simulink model "claw_machine_design_sofia"  (R2022b)
settings: Solver=VariableStepAuto  StartTime=0.0  StopTime=inf  RelTol=1e-3
libraries: vrlib x1
settings Model: Creator=Sofia  LastModifiedBy=Sofia

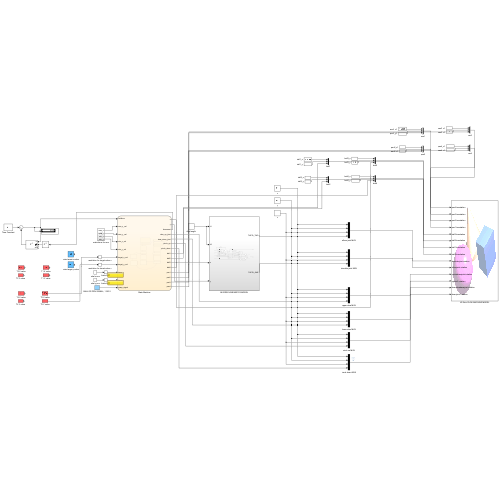
[thumbnail: Simulink's stored preview of the top-level diagram]
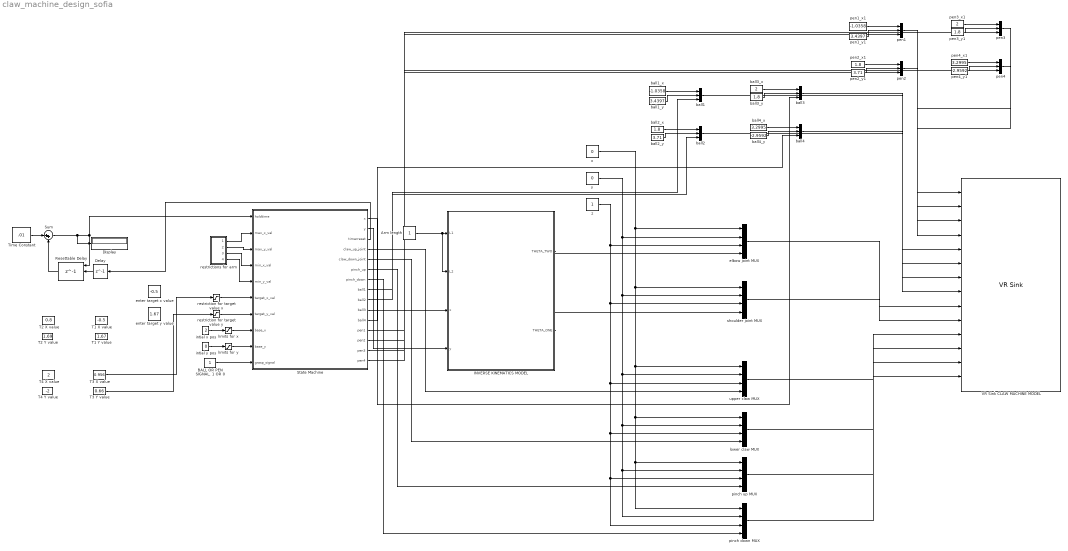
== system claw_machine_design_sofia ==
  Arm length : Constant
  "BALL OR PEN SIGNAL, 1 OR 0" : Constant
  Delay : Delay  DelayLength=1  InitialCondition=0
  Display : Display
  INVERSE KINEMATICS MODEL : Subsystem  Description=Calculates joint angles based on end effector x and y positions
  Resettable Delay : Delay  DelayLength=1  InitialConditionSource=Input port  ExternalReset=Rising
      settings: InputPortMap=u0,r5,p4
  State Machine : Stateflow chart  TreatAsAtomicUnit=on
  Sum : Sum  Inputs=|++
  T1 X value : Constant  Value=-0.5
  T1 Y value : Constant  Value=1.67
  T2 X value : Constant  Value=0.8
  T2 Y value : Constant  Value=1.69
  T3 X value : Constant  Value=0.956
  T3 Y value : Constant  Value=0.66
  T4 X value : Constant  Value=2
  T4 Y value : Constant  Value=-2
  Time Constant : Constant  Value=.01
  VR Sink CLAW MACHINE MODEL : vrlib/VR Sink  InstantiateOnLoad=on  SampleTime=0.1  ViewEnable=on  RemoteChange=off  RemoteView=off  FieldsWritten=pen4.translation.3.1.1.double#pen3.translation.3.1.1.double#pen2.translation.3.1.1.double#pen1.translation.3.1.1.double#ball3.translation.3.1.1.double#ball2.translation.3.1.1.double#ball1.translation.3.1.1.double#ball4.translation.3.1.1.double#shoulderjoint.rotation.4.1.1.double#elbowjoint.rotation.4.1.1.double#upclawbasejoint.rotation.4.1.1.double#upjoint1.rotation.4.1.1.double#downclawbasejoint.rotation.4.1.1.double#downjoint1.rotation.4.1.1.double  WorldFileName=C:\Users\Sofia\OneDrive\Semester 4\691 Brain Computer Interfaces\FINAL PROJECT BCI\clawmachinemodel.wrl  AutoView=off  VideoDimensions=[]  AllowVariableSize=off
  ball{1..4} (4 alike) : Mux  Inputs=3
  ball1_x : Constant  Value=-1.0358
  ball1_y : Constant  Value=3.4397
  ball2_x : Constant  Value=1.8
  ball2_y : Constant  Value=3.71
  ball3_x : Constant  Value=2
  ball3_y : Constant  Value=1.8
  ball4_x : Constant  Value=3.2995
  ball4_y : Constant  Value=-2.9592
  elbow joint MUX : Mux
  enter target x value : Constant  Value=-0.5
  enter target y value : Constant  Value=1.67
  intial x pos : Constant  Value=2
  intial y pos : Constant  Value=0
  limits for x : Saturate  UpperLimit=2  LowerLimit=0
  limits for y : Saturate  UpperLimit=2  LowerLimit=0
  lower claw MUX : Mux
  pen{1..4} (4 alike) : Mux  Inputs=3
  pen1_x1 : Constant  Value=-1.0358
  pen1_y1 : Constant  Value=3.4397
  pen2_x1 : Constant  Value=1.8
  pen2_y1 : Constant  Value=3.71
  pen3_x1 : Constant  Value=2
  pen3_y1 : Constant  Value=1.8
  pen4_x1 : Constant  Value=3.2995
  pen4_y1 : Constant  Value=-2.9592
  pinch down MUX : Mux
  pinch up MUX : Mux
  restriction for target value x : Saturate  UpperLimit=2
  restriction for target value y : Saturate  UpperLimit=2  LowerLimit=-2
  restrictions for arm : Subsystem
  shoulder joint MUX : Mux
  upper claw MUX : Mux
  x : Constant  Value=0
  y : Constant  Value=0
  z : Constant
  wires:
  State Machine/3(timerreset) -> Delay/1
  Resettable Delay/1 -> Sum/2
  x/1 -> shoulder joint MUX/1, upper claw MUX/1, lower claw MUX/1, pinch up MUX/1, pinch down MUX/1, elbow joint MUX/1
  z/1 -> elbow joint MUX/3, shoulder joint MUX/3, upper claw MUX/3, pinch down MUX/3, pinch up MUX/3, lower claw MUX/3
  y/1 -> elbow joint MUX/2, shoulder joint MUX/2, upper claw MUX/2, pinch up MUX/2, pinch down MUX/2, lower claw MUX/2
  Sum/1 -> State Machine/1(holdtime), Resettable Delay/1, Display/1
  Time Constant/1 -> Sum/1
  Delay/1 -> Resettable Delay/2
  Arm length/1 -> INVERSE KINEMATICS MODEL/2(L2), INVERSE KINEMATICS MODEL/1(L1)
  INVERSE KINEMATICS MODEL/2(THETA_ONE) -> shoulder joint MUX/4
  INVERSE KINEMATICS MODEL/1(THETA_TWO) -> elbow joint MUX/4
  State Machine/1(x) -> INVERSE KINEMATICS MODEL/3(x)
  State Machine/2(y) -> INVERSE KINEMATICS MODEL/4(y)
  restrictions for arm/1(max_x) -> State Machine/2(max_x_val)
  restrictions for arm/2(max_y) -> State Machine/3(max_y_val)
  restrictions for arm/3(min_x) -> State Machine/4(min_x_val)
  restrictions for arm/4(min_y) -> State Machine/5(min_y_val)
  restriction for target value x/1 -> State Machine/6(target_x_val)
  restriction for target value y/1 -> State Machine/7(target_y_val)
  "BALL OR PEN SIGNAL, 1 OR 0"/1 -> State Machine/10(grasp_signal)
  ball4_x/1 -> ball4/1
  ball4_y/1 -> ball4/2
  ball1_x/1 -> ball1/1
  ball1_y/1 -> ball1/2
  ball3_x/1 -> ball3/1
  ball3_y/1 -> ball3/2
  ball2_y/1 -> ball2/2
  ball2_x/1 -> ball2/1
  State Machine/4(claw_up_joint) -> upper claw MUX/4
  State Machine/5(claw_down_joint) -> lower claw MUX/4
  State Machine/6(pinch_up) -> pinch up MUX/4
  State Machine/7(pinch_down) -> pinch down MUX/4
  State Machine/8(ball1) -> ball1/3
  State Machine/9(ball2) -> ball2/3
  State Machine/10(ball3) -> ball3/3
  State Machine/11(ball4) -> ball4/3
  ball4/1 -> VR Sink CLAW MACHINE MODEL/8
  ball3/1 -> VR Sink CLAW MACHINE MODEL/5
  ball2/1 -> VR Sink CLAW MACHINE MODEL/6
  ball1/1 -> VR Sink CLAW MACHINE MODEL/7
  shoulder joint MUX/1 -> VR Sink CLAW MACHINE MODEL/9
  elbow joint MUX/1 -> VR Sink CLAW MACHINE MODEL/10
  upper claw MUX/1 -> VR Sink CLAW MACHINE MODEL/11
  pinch up MUX/1 -> VR Sink CLAW MACHINE MODEL/12
  lower claw MUX/1 -> VR Sink CLAW MACHINE MODEL/13
  pinch down MUX/1 -> VR Sink CLAW MACHINE MODEL/14
  pen2_x1/1 -> pen2/1
  pen2_y1/1 -> pen2/2
  pen3_y1/1 -> pen3/2
  pen3_x1/1 -> pen3/1
  pen1_y1/1 -> pen1/2
  pen1_x1/1 -> pen1/1
  pen4_y1/1 -> pen4/2
  pen4_x1/1 -> pen4/1
  pen1/1 -> VR Sink CLAW MACHINE MODEL/4
  pen2/1 -> VR Sink CLAW MACHINE MODEL/3
  pen3/1 -> VR Sink CLAW MACHINE MODEL/2
  pen4/1 -> VR Sink CLAW MACHINE MODEL/1
  State Machine/12(pen1) -> pen1/3
  State Machine/13(pen2) -> pen2/3
  State Machine/14(pen3) -> pen3/3
  State Machine/15(pen4) -> pen4/3
  T3 X value/1 -> restriction for target value x/1
  T3 Y value/1 -> restriction for target value y/1
  intial x pos/1 -> limits for x/1
  intial y pos/1 -> limits for y/1
  limits for x/1 -> State Machine/8(base_x)
  limits for y/1 -> State Machine/9(base_y)

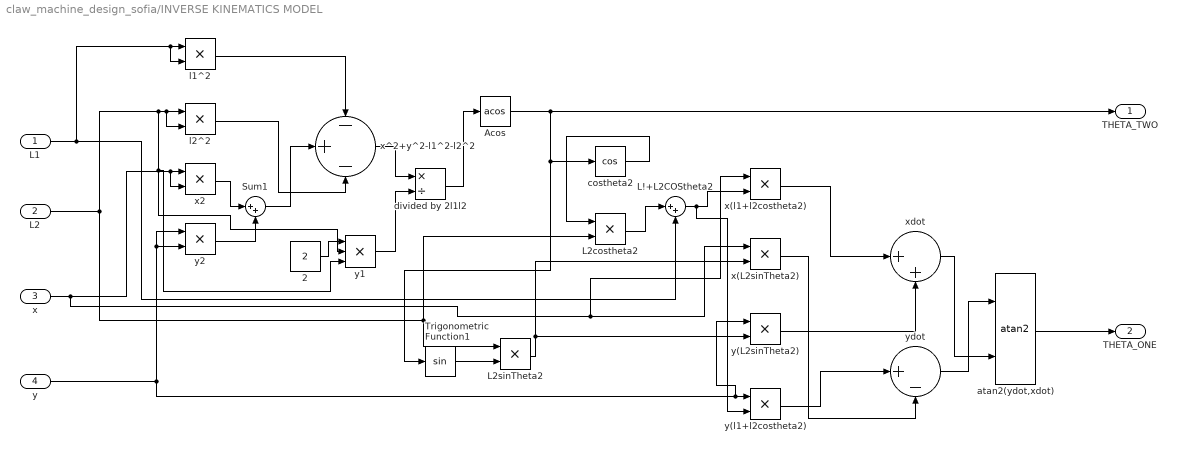
== system claw_machine_design_sofia/INVERSE KINEMATICS MODEL ==
  L1 : Inport
  L2 : Inport  Port=2
  x : Inport  Port=3
  y : Inport  Port=4
  2 : Constant  Value=2
  Acos : Trigonometry  Operator=acos
  L!+L2COStheta2 : Sum  Inputs=|++
  L2costheta2 : Product
  L2sinTheta2 : Product
  Sum1 : Sum  Inputs=|++
  Trigonometric Function1 : Trigonometry
  atan2(ydot,xdot) : Trigonometry  Operator=atan2
  costheta2 : Trigonometry  Operator=cos
  divided by 2l1l2 : Product  Inputs=*/
  l1^2 : Product
  l2^2 : Product
  x(L2sinTheta2) : Product
  x(l1+l2costheta2) : Product
  x2 : Product
  x^2+y^2-l1^2-l2^2 : Sum  Inputs=-+-
  xdot : Sum  Inputs=|++
  y(L2sinTheta2) : Product
  y(l1+l2costheta2) : Product
  y1 : Product  Inputs=3
  y2 : Product
  ydot : Sum  Inputs=|+-
  THETA_TWO : Outport
  THETA_ONE : Outport  Port=2
  wires:
  x2/1 -> Sum1/1
  Sum1/1 -> x^2+y^2-l1^2-l2^2/2
  y/1 -> y(L2sinTheta2)/1, y(l1+l2costheta2)/1, y2/2, y2/1
  x(L2sinTheta2)/1 -> ydot/2
  atan2(ydot,xdot)/1 -> THETA_ONE/1
  x/1 -> x(l1+l2costheta2)/1, x(L2sinTheta2)/1, x2/2, x2/1
  L2/1 -> L2sinTheta2/1, L2costheta2/2, y1/3, y1/2, l2^2/2, l2^2/1
  Trigonometric Function1/1 -> L2sinTheta2/2
  L!+L2COStheta2/1 -> y(l1+l2costheta2)/2, x(l1+l2costheta2)/2
  Acos/1 -> THETA_TWO/1, Trigonometric Function1/1, costheta2/1
  y(L2sinTheta2)/1 -> xdot/2
  l2^2/1 -> x^2+y^2-l1^2-l2^2/3
  2/1 -> y1/1
  divided by 2l1l2/1 -> Acos/1
  l1^2/1 -> x^2+y^2-l1^2-l2^2/1
  xdot/1 -> atan2(ydot,xdot)/2
  L1/1 -> L!+L2COStheta2/2, l1^2/2, l1^2/1
  y2/1 -> Sum1/2
  y(l1+l2costheta2)/1 -> ydot/1
  ydot/1 -> atan2(ydot,xdot)/1
  L2sinTheta2/1 -> x(L2sinTheta2)/2, y(L2sinTheta2)/2
  x^2+y^2-l1^2-l2^2/1 -> divided by 2l1l2/1
  y1/1 -> divided by 2l1l2/2
  L2costheta2/1 -> L!+L2COStheta2/1
  x(l1+l2costheta2)/1 -> xdot/1
  costheta2/1 -> L2costheta2/1

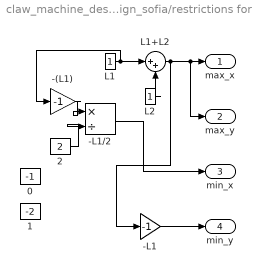
== system claw_machine_design_sofia/restrictions for arm ==
  -(L1) : Gain  Gain=-1
  -L1 : Gain  Gain=-1
  -L1/2 : Product  Inputs=*/
  0 : Constant  Value=-1
  1 : Constant  Value=-2
  2 : Constant  Value=2
  L1 : Constant
  L1+L2 : Sum  Inputs=|++
  L2 : Constant
  max_x : Outport
  max_y : Outport  Port=2
  min_x : Outport  Port=3
  min_y : Outport  Port=4
  wires:
  L1+L2/1 -> -L1/1, max_y/1, max_x/1
  L1/1 -> -(L1)/1, L1+L2/1
  L2/1 -> L1+L2/2
  -L1/1 -> min_y/1
  -(L1)/1 -> -L1/2/1
  2/1 -> -L1/2/2
  -L1/2/1 -> min_x/1

== stateflow chart claw_machine_design_sofia/State Machine ==
  state basestate
    if base_x > 2
    x = 2;
    elseif base_x < -1
    x = -1;
    else
    x = base_x;
    end
    if base_y > 2
    y = 2;
    elseif base_y < -2
    y = -2;
    else
    y = base_y;
    end
    claw_up_joint=0.5; claw_down_joint=-0.5; pinch_up=0; pinch_down=0;
    ball1=0; ball2=0; ball3=0; ball4=0; pen1=0; pen2=0; pen3=0; pen4=0;
    timerreset=0;
  state resetstate
    x=x; y=y; claw_up_joint=claw_up_joint; claw_down_joint=claw_down_joint; pinch_up=pinch_up; pinch_down=pinch_down;
    ball1=ball1; ball2=ball2; ball3=ball3; ball4=ball4; pen1=pen1; pen2=pen2; pen3=pen3; pen4=pen4; timerreset=1;
  state holdstate1
    x=x; y=y; claw_up_joint=claw_up_joint; claw_down_joint=claw_down_joint;
    pinch_up=pinch_up; pinch_down=pinch_down; ball1=ball1; ball2=ball2; ball3=ball3; ball4=ball4;
    pen1=pen1; pen2=pen2; pen3=pen3; pen4=pen4; timerreset=0;
  state holdstate
    x=base_x; y=base_y; claw_up_joint=0.5; claw_down_joint=-0.5; pinch_up=0; pinch_down=0;
    ball1=0; ball2=0; ball3=0; ball4=0; pen1=0; pen2=0; pen3=0; pen4=0;
    timerreset=0;
  state basestateback
    x=base_x; y=base_y; claw_up_joint=0.5; claw_down_joint=-0.5; pinch_up=0; pinch_down=0;
    ball1=0; ball2=0; ball3=0; ball4=0; pen1=0; pen2=0; pen3=0; pen4=0; timerreset=0;
  state transitiontotargetstate
    if (x <  target_x_val && x < max_x_val)
    x = x + 0.01;
    end
    if (x > target_x_val && x > min_x_val)
    x = x - 0.01;
    end
    if (y <  target_y_val && y < max_y_val)
    y = y + 0.01;
    end
    if (y > target_y_val && y > min_y_val)
    y = y - 0.01;
    end
    claw_up_joint=claw_up_joint;
    claw_down_joint=claw_down_joint;
    pinch_up=pinch_up; pinch_down=pinch_down;
    ball1=0; ball2=0; ball3=0; ball4=0;
    pen1=0; pen2=0; pen3=0; pen4=0;
    timerreset=0;
  state transitiontobasestate
    if (x > base_x && x > min_x_val)
    x = x - 0.01;
    end
    if (x < base_x && x < max_x_val)
    x = x + 0.01;
    end
    if (y > base_y && y > min_y_val)
    y = y - 0.02;
    end
    if (y < base_y && y < max_y_val)
    y = y + 0.02;
    end
    claw_up_joint=claw_up_joint;
    claw_down_joint=claw_down_joint;
    pinch_up=pinch_up; pinch_down=pinch_down;
    ball1=ball1; ball2=ball2; ball3=ball3; ball4=ball4;
    pen1=pen1; pen2=pen2; pen3=pen3; pen4=pen4;
    timerreset=0;
  state targetstate
    x=target_x_val; y=target_y_val;
    claw_up_joint=claw_up_joint; claw_down_joint=claw_down_joint;
    pinch_up=pinch_up; pinch_down=pinch_down;
    ball1=0; ball2=0; ball3=0; ball4=0;
    pen1=0; pen2=0; pen3=0; pen4=0;
    timerreset=0;
  state ungrabstate
    x=target_x_val;y=target_y_val;
    claw_up_joint=0.5; claw_down_joint=-0.5; pinch_up=0; pinch_down=0;
    ball1=ball1; ball2=ball2; ball3=ball3; ball4=ball4;
    pen1=pen1; pen2=pen2; pen3=pen3; pen4=pen4; timerreset=0;
  state transitiontopinchstate
    x=target_x_val;y=target_y_val;
    if claw_up_joint > -0.1
    claw_up_joint = claw_up_joint-0.01
    end
    if claw_down_joint < 0.1
    claw_down_joint = claw_down_joint+0.01
    end
    if pinch_up > -0.33
    pinch_up = pinch_up - 0.01
    end
    if pinch_down < 0.33
    pinch_down = pinch_down +0.01
    end
    pen1=0; pen2=0; pen3=0; pen4=0;
    ball1=100; ball2=100; ball3=100; ball4=100;
    timerreset=0;
  state transitiontograbstate
    x=target_x_val;y=target_y_val;
    if claw_up_joint > 0.3
    claw_up_joint = claw_up_joint-0.001
    end
    if claw_down_joint < -0.3
    claw_down_joint = claw_down_joint+0.001
    end
    if pinch_up > -0.1
    pinch_up = pinch_up - 0.001
    end
    if pinch_down < 0.1
    pinch_down = pinch_down +0.001
    end
    ball1=0; ball2=0; ball3=0; ball4=0;
    pen1=100; pen2=100; pen3=100; pen4=100;
    timerreset=0;
  state transitiontoungrabstate
    x=target_x_val;y=target_y_val;
    if claw_up_joint < 0.5
    claw_up_joint = claw_up_joint + 0.001
    end
    if claw_down_joint > -0.5
    claw_down_joint = claw_down_joint - 0.001
    end
    if pinch_up < 0
    pinch_up = pinch_up + 0.001
    end
    if pinch_down > 0
    pinch_down = pinch_down - 0.001
    end
    ball1=ball1; ball2=ball2; ball3=ball3; ball4=ball4;
    pen1=pen1; pen2=pen2; pen3=pen3; pen4=pen4;
    timerreset=0;
  state grabstate
    x=target_x_val;y=target_y_val;
    claw_up_joint=0.3; claw_down_joint=-0.3;
    pinch_up = -0.1; pinch_down=0.1;
    if target_x_val==-0.5 && target_y_val==1.67
    ball1=0; ball2=100; ball3=100; ball4=100;
    elseif target_x_val==0.8 && target_y_val==1.69
    ball1=100; ball2=0; ball3=100; ball4=100;
    elseif target_x_val==0.956 && target_y_val==0.66
    ball1=100; ball2=100; ball3=0; ball4=100;
    elseif target_x_val==2 && target_y_val==-2
    ball1=100; ball2=100; ball3=100; ball4=0;
    else
    ball1=0; ball2=0; ball3=0; ball4=0;
    end
    pen1=100; pen2=100; pen3=100; pen4=100;
    timerreset=0;
  state pinchstate
    x=target_x_val;y=target_y_val;
    claw_up_joint=-0.1; claw_down_joint=0.1;
    pinch_up = -0.33; pinch_down=0.33;
    if target_x_val==-0.5 && target_y_val==1.67
    pen1=0; pen2=100; pen3=100; pen4=100;
    elseif target_x_val==0.8 && target_y_val==1.69
    pen1=100; pen2=0; pen3=100; pen4=100;
    elseif target_x_val==0.956 && target_y_val==0.66
    pen1=100; pen2=100; pen3=0; pen4=100;
    elseif target_x_val==2 && target_y_val==-2
    pen1=100; pen2=100; pen3=100; pen4=0;
    else
    pen1=0; pen2=0; pen3=0; pen4=0;
    end
    ball1=100; ball2=100; ball3=100; ball4=100;
    timerreset=0;
  state holdaftergrabstate
    x=x; y=y; claw_up_joint=claw_up_joint; claw_down_joint=claw_down_joint;
    pinch_up=pinch_up; pinch_down=pinch_down;
    ball1=ball1; ball2=ball2; ball3=ball3; ball4=ball4;
    pen1=pen1; pen2=pen2; pen3=pen3; pen4=pen4;
    timerreset=0;
  (default) -> basestate
  resetstate -> holdstate
  holdstate1 -> resetstate : [holdtime > 26]
  basestate -> holdstate : [holdtime > 2]
  basestateback -> holdstate1 : [holdtime > 25]
  holdstate -> transitiontotargetstate : [holdtime > 4]
  transitiontobasestate -> basestateback : [abs(x - base_x) <= 0.02 && abs(y - base_y) <= 0.02]
  transitiontotargetstate -> targetstate : [abs(x - target_x_val) <= 0.02 && abs(y - target_y_val) <= 0.02]
  ungrabstate -> transitiontobasestate : [holdtime > 20]
  targetstate -> transitiontopinchstate [order 1] : [holdtime > 8 && grasp_signal == 0]
  targetstate -> transitiontograbstate [order 2] : [holdtime>8 && grasp_signal==1]
  transitiontoungrabstate -> ungrabstate : [claw_up_joint >= 0.5 && claw_down_joint <= -0.5 && pinch_up >=0 && pinch_down <= 0 ]
  transitiontopinchstate -> pinchstate : [abs(claw_up_joint - (-0.1)) <= 0.01 && abs(claw_down_joint - (0.1)) <= 0.01 && abs(pinch_up - (-0.33)) <= 0.01 && abs(pinch_down - 0.33) <= 0.01]
  transitiontograbstate -> grabstate : [abs(claw_up_joint - (0.3)) <= 0.01 && abs(claw_down_joint - (-0.3)) <= 0.01 && abs(pinch_up - (-0.1)) <= 0.01 && abs(pinch_down - 0.1) <= 0.01]
  holdaftergrabstate -> transitiontoungrabstate : [holdtime > 15]
  grabstate -> holdaftergrabstate : [holdtime > 13]
  pinchstate -> holdaftergrabstate : [holdtime > 13]
  data: holdtime input; x output; y output; timerreset output; claw_up_joint output; claw_down_joint output; max_x_val input; max_y_val input; min_x_val input; min_y_val input; target_x_val input; target_y_val input; base_x input; base_y input; pinch_up output; pinch_down output; grasp_signal input; ball1 output; ball2 output; ball3 output; ball4 output; pen1 output; pen2 output; pen3 output; pen4 output
